simulink library "ComponentLibrary"  (R2017b)
settings: Solver=VariableStepAuto  StartTime=0.0  StopTime=10.0  RelTol=1e-3
undefined symbols (not defined in the file): pelvisPosition, pelvisVelocity, X, Y, Z
libraries: xpcethercatlib x79, sm_lib x21, nesl_utility x13, slrtlib x3, ComponentLibrary x2
(part 1 of 2)
settings Model: Creator=Mikhail  LastModifiedBy=jreher

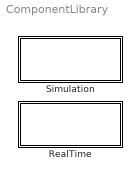
== system ComponentLibrary ==
  RealTime : Subsystem
  Simulation : Subsystem

== system ComponentLibrary/RealTime ==
  Battery : Subsystem
      mask Display: image('Battery.png');
  Elmo Drive : Subsystem  mask{ethercatName=Drive (Elmo Drive), slaveAddress=0, gearRatio=1, torqueConstant=1, encoderCounts=2^13, peakCurrentLimit=0}
      mask prompts: ethercatName "EtherCAT Name:"; slaveAddress "Slave Address"; gearRatio "Gear Ratio:"; torqueConstant "Torque Constant:"; encoderCounts "Encoder Counts:"; peakCurrentLimit "Peak Current Limit:"
      mask init:
      | % Set PDO transmit
      | set_param([gcb '/Mode of Operation PDO Transmit'], 'sig_name', [ethercatName '.Outputs.Mode of operation']);
      | set_param([gcb '/Target Torque PDO Transmit'], 'sig_name', [ethercatName '.Outputs.Target Torque']);
      | set_param([gcb '/Control Word PDO Transmit'], 'sig_name', [ethercatName '.Outputs.Control word']);
      | 
      | % Set PDO receive
      | set_param([gcb '/Status Word PDO Receive'], 'sig_name', [ethercatName '.Inputs.Status word']);
      | set_param([gcb '/Position Actual PDO Receive'], 'sig_name', [ethercatName '.Inputs.Position actual value']);
      | set_param([gcb '/Velocity Actual PDO Receive'], 'sig_name', [ethercatName '.Inputs.Velocity actual value']);
      | set_param([gcb '/Torque Actual PDO Receive'], 'sig_name', [ethercatName '.Inputs.Torque actual value']);
      | set_param([gcb '/DC Link Voltage PDO Receive'], 'sig_name', [ethercatName '.Inputs.DC link circuit voltage']);
      | 
      | % Set SDO temperature upload
      | set_param([gcb '/Drive Temperature Sync SDO Upload'], 'index', '8867');
      | set_param([gcb '/Drive Temperature Sync SDO Upload'], 'subIndex', '1');
      | set_param([gcb '/Drive Temperature Sync SDO Upload'], 'slave_name', ethercatName);
      | set_param([gcb '/Drive Temperature Sync SDO Upload'], 'slave_addr', num2str(slaveAddress));
      | set_param([gcb '/Drive Temperature Sync SDO Upload'], 'slave_found', '1');
      | 
      | % Set SDO Current limit upload
      | set_param([gcb '/Current Limit Sync SDO Upload'], 'index', '12351');
      | set_param([gcb '/Current Limit Sync SDO Upload'], 'subIndex', '1');
      | set_param([gcb '/Current Limit Sync SDO Upload'], 'slave_name', ethercatName);
      | set_param([gcb '/Current Limit Sync SDO Upload'], 'slave_addr', num2str(slaveAddress));
      | set_param([gcb '/Current Limit Sync SDO Upload'], 'slave_found', '1');
      mask Display: image('Elmo Drive.png')
  Radio : Subsystem
      mask Display: image('Radio.png');
  Target PC : Subsystem  mask{config_file=, pci_bus=0, pci_slot=0, pci_function=0}
      mask prompts: config_file "EtherCAT configuration file:"; pci_bus "PCI bus:"; pci_slot "PCI slot:"; pci_function "PCI function:"
      mask TypeOptions config_file: EtherCAT Init/config_file
      mask TypeOptions pci_bus: EtherCAT Init/pci_bus
      mask TypeOptions pci_slot: EtherCAT Init/pci_slot
      mask TypeOptions pci_function: EtherCAT Init/pci_function
  VectorNav : Subsystem  mask{preRotationMatrix=eye(3), postRotationMatrix=eye(3)}
      mask prompts: preRotationMatrix "Pre Rotation Matrix:"; postRotationMatrix "Post Rotation Matrix:"
      mask Display: image('VectorNav.png')

== system ComponentLibrary/Simulation ==
  Battery : Subsystem
      mask Display: image('Battery.png');
  Elmo Drive : Subsystem  mask{gearRatio=25, rotorInertia=0.000061, encoderResolution=2^13, peakTorque=4.5, peakSpeed=2900*(2*pi/60), initialPosition=0, initialVelocity=0}
      mask prompts: gearRatio "Gear Ratio:"; rotorInertia "Motor rotor inertia (kg*m^2):"; encoderResolution "Input Encoder Resolution (ticks/rev):"; peakTorque "Peak torque of motor (N*m):"; peakSpeed "Peak speed of motor (rad/s):"; initialPosition "Initial Position (rad):"; initialVelocity "Initial Velocity (rad/s):"
      mask Display: image('Elmo Drive.png');
  Radio : Subsystem
      mask Display: image('Radio.png');
  Target PC : Subsystem
  VectorNav : Subsystem  mask{preRotationMatrix=eye(3), postRotationMatrix=eye(3)}
      mask prompts: preRotationMatrix "Pre Rotation Matrix:"; postRotationMatrix "Post Rotation Matrix"
      mask Display: image('VectorNav.png');
  World : Subsystem

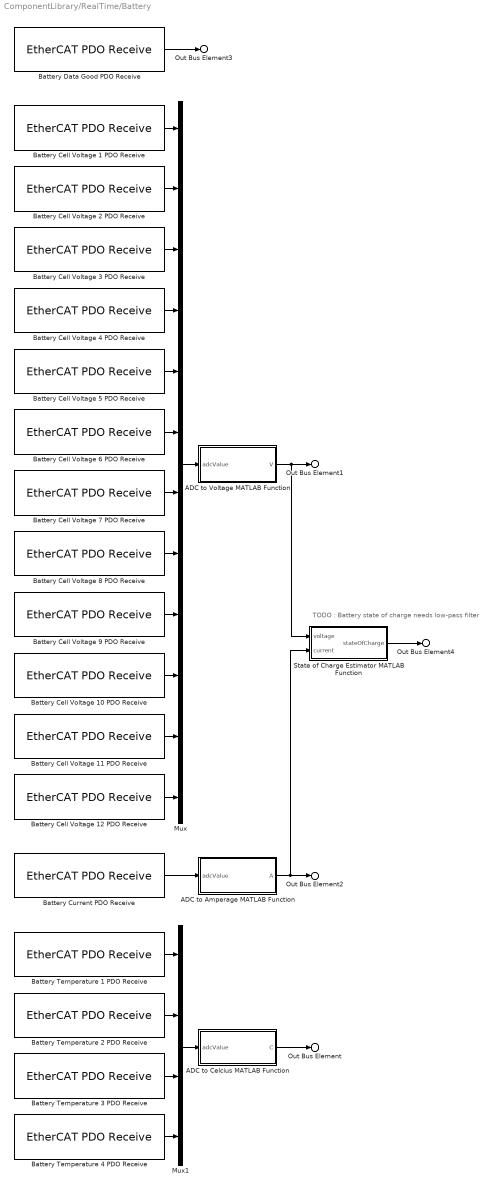
== system ComponentLibrary/RealTime/Battery ==
  note: TODO : Battery state of charge needs low-pass filter
  ADC to Amperage MATLAB Function : MATLAB Function  TreatAsAtomicUnit=on
  ADC to Celcius MATLAB Function : MATLAB Function  TreatAsAtomicUnit=on
  ADC to Voltage MATLAB Function : MATLAB Function  TreatAsAtomicUnit=on
  Battery Cell Voltage 1 PDO Receive : xpcethercatlib/EtherCAT PDO Receive  Priority=2  sig_name=Pelvis Medulla.BMS Inputs.Cell Voltage 01  sig_offset=1608  sig_type=uint16  type_size=16  sig_dim=1  device_id=0  sample_time=0.000500
      settings: SourceProductName=Simulink Real-Time  SourceProductBaseCode=XP
  Battery Cell Voltage 10 PDO Receive : xpcethercatlib/EtherCAT PDO Receive  Priority=2  sig_name=Pelvis Medulla.BMS Inputs.Cell Voltage 10  sig_offset=1752  sig_type=uint16  type_size=16  sig_dim=1  device_id=0  sample_time=0.000500
      settings: SourceProductName=Simulink Real-Time  SourceProductBaseCode=XP
  Battery Cell Voltage 11 PDO Receive : xpcethercatlib/EtherCAT PDO Receive  Priority=2  sig_name=Pelvis Medulla.BMS Inputs.Cell Voltage 11  sig_offset=1768  sig_type=uint16  type_size=16  sig_dim=1  device_id=0  sample_time=0.000500
      settings: SourceProductName=Simulink Real-Time  SourceProductBaseCode=XP
  Battery Cell Voltage 12 PDO Receive : xpcethercatlib/EtherCAT PDO Receive  Priority=2  sig_name=Pelvis Medulla.BMS Inputs.Cell Voltage 12  sig_offset=1784  sig_type=uint16  type_size=16  sig_dim=1  device_id=0  sample_time=0.000500
      settings: SourceProductName=Simulink Real-Time  SourceProductBaseCode=XP
  Battery Cell Voltage 2 PDO Receive : xpcethercatlib/EtherCAT PDO Receive  Priority=2  sig_name=Pelvis Medulla.BMS Inputs.Cell Voltage 02  sig_offset=1624  sig_type=uint16  type_size=16  sig_dim=1  device_id=0  sample_time=0.000500
      settings: SourceProductName=Simulink Real-Time  SourceProductBaseCode=XP
  Battery Cell Voltage 3 PDO Receive : xpcethercatlib/EtherCAT PDO Receive  Priority=2  sig_name=Pelvis Medulla.BMS Inputs.Cell Voltage 03  sig_offset=1640  sig_type=uint16  type_size=16  sig_dim=1  device_id=0  sample_time=0.000500
      settings: SourceProductName=Simulink Real-Time  SourceProductBaseCode=XP
  Battery Cell Voltage 4 PDO Receive : xpcethercatlib/EtherCAT PDO Receive  Priority=2  sig_name=Pelvis Medulla.BMS Inputs.Cell Voltage 04  sig_offset=1656  sig_type=uint16  type_size=16  sig_dim=1  device_id=0  sample_time=0.000500
      settings: SourceProductName=Simulink Real-Time  SourceProductBaseCode=XP
  Battery Cell Voltage 5 PDO Receive : xpcethercatlib/EtherCAT PDO Receive  Priority=2  sig_name=Pelvis Medulla.BMS Inputs.Cell Voltage 05  sig_offset=1672  sig_type=uint16  type_size=16  sig_dim=1  device_id=0  sample_time=0.000500
      settings: SourceProductName=Simulink Real-Time  SourceProductBaseCode=XP
  Battery Cell Voltage 6 PDO Receive : xpcethercatlib/EtherCAT PDO Receive  Priority=2  sig_name=Pelvis Medulla.BMS Inputs.Cell Voltage 06  sig_offset=1688  sig_type=uint16  type_size=16  sig_dim=1  device_id=0  sample_time=0.000500
      settings: SourceProductName=Simulink Real-Time  SourceProductBaseCode=XP
  Battery Cell Voltage 7 PDO Receive : xpcethercatlib/EtherCAT PDO Receive  Priority=2  sig_name=Pelvis Medulla.BMS Inputs.Cell Voltage 07  sig_offset=1704  sig_type=uint16  type_size=16  sig_dim=1  device_id=0  sample_time=0.000500
      settings: SourceProductName=Simulink Real-Time  SourceProductBaseCode=XP
  Battery Cell Voltage 8 PDO Receive : xpcethercatlib/EtherCAT PDO Receive  Priority=2  sig_name=Pelvis Medulla.BMS Inputs.Cell Voltage 08  sig_offset=1720  sig_type=uint16  type_size=16  sig_dim=1  device_id=0  sample_time=0.000500
      settings: SourceProductName=Simulink Real-Time  SourceProductBaseCode=XP
  Battery Cell Voltage 9 PDO Receive : xpcethercatlib/EtherCAT PDO Receive  Priority=2  sig_name=Pelvis Medulla.BMS Inputs.Cell Voltage 09  sig_offset=1736  sig_type=uint16  type_size=16  sig_dim=1  device_id=0  sample_time=0.000500
      settings: SourceProductName=Simulink Real-Time  SourceProductBaseCode=XP
  Battery Current PDO Receive : xpcethercatlib/EtherCAT PDO Receive  Priority=2  sig_name=Pelvis Medulla.BMS Inputs.Current  sig_offset=1864  sig_type=uint16  type_size=16  sig_dim=1  device_id=0  sample_time=0.000500
      settings: SourceProductName=Simulink Real-Time  SourceProductBaseCode=XP
  Battery Data Good PDO Receive : xpcethercatlib/EtherCAT PDO Receive  Priority=2  sig_name=Pelvis Medulla.BMS Inputs.Battery Data Good  sig_offset=1816  sig_type=boolean  type_size=1  sig_dim=1  device_id=0  sample_time=0.0005
      settings: SourceProductName=Simulink Real-Time  SourceProductBaseCode=XP
  Battery Temperature 1 PDO Receive : xpcethercatlib/EtherCAT PDO Receive  Priority=2  sig_name=Pelvis Medulla.BMS Inputs.Temperature 1  sig_offset=1800  sig_type=uint16  type_size=16  sig_dim=1  device_id=0  sample_time=0.000500
      settings: SourceProductName=Simulink Real-Time  SourceProductBaseCode=XP
  Battery Temperature 2 PDO Receive : xpcethercatlib/EtherCAT PDO Receive  Priority=2  sig_name=Pelvis Medulla.BMS Inputs.Temperature 2  sig_offset=1816  sig_type=uint16  type_size=16  sig_dim=1  device_id=0  sample_time=0.000500
      settings: SourceProductName=Simulink Real-Time  SourceProductBaseCode=XP
  Battery Temperature 3 PDO Receive : xpcethercatlib/EtherCAT PDO Receive  Priority=2  sig_name=Pelvis Medulla.BMS Inputs.Temperature 3  sig_offset=1832  sig_type=uint16  type_size=16  sig_dim=1  device_id=0  sample_time=0.000500
      settings: SourceProductName=Simulink Real-Time  SourceProductBaseCode=XP
  Battery Temperature 4 PDO Receive : xpcethercatlib/EtherCAT PDO Receive  Priority=2  sig_name=Pelvis Medulla.BMS Inputs.Temperature 4  sig_offset=1848  sig_type=uint16  type_size=16  sig_dim=1  device_id=0  sample_time=0.000500
      settings: SourceProductName=Simulink Real-Time  SourceProductBaseCode=XP
  Mux : Mux  Inputs=12
  Mux1 : Mux
  State of Charge Estimator MATLAB Function : MATLAB Function  TreatAsAtomicUnit=on
  Out Bus Element3 : Outport  PortName=OutBus  Element=dataGood
  Out Bus Element4 : Outport  PortName=OutBus  Element=stateOfCharge
  Out Bus Element1 : Outport  PortName=OutBus  Element=voltage
  Out Bus Element2 : Outport  PortName=OutBus  Element=current
  Out Bus Element : Outport  PortName=OutBus  Element=temperature
  wires:
  Battery Temperature 1 PDO Receive/1 -> Mux1/1
  Battery Temperature 2 PDO Receive/1 -> Mux1/2
  Battery Temperature 3 PDO Receive/1 -> Mux1/3
  Battery Temperature 4 PDO Receive/1 -> Mux1/4
  Battery Cell Voltage 1 PDO Receive/1 -> Mux/1
  Battery Cell Voltage 2 PDO Receive/1 -> Mux/2
  Battery Cell Voltage 3 PDO Receive/1 -> Mux/3
  Battery Cell Voltage 4 PDO Receive/1 -> Mux/4
  Battery Cell Voltage 5 PDO Receive/1 -> Mux/5
  Battery Cell Voltage 6 PDO Receive/1 -> Mux/6
  Battery Cell Voltage 7 PDO Receive/1 -> Mux/7
  Battery Cell Voltage 8 PDO Receive/1 -> Mux/8
  Battery Cell Voltage 9 PDO Receive/1 -> Mux/9
  Battery Cell Voltage 10 PDO Receive/1 -> Mux/10
  Battery Cell Voltage 11 PDO Receive/1 -> Mux/11
  Battery Cell Voltage 12 PDO Receive/1 -> Mux/12
  Mux/1 -> ADC to Voltage MATLAB Function/1(adcValue)
  Battery Current PDO Receive/1 -> ADC to Amperage MATLAB Function/1(adcValue)
  ADC to Celcius MATLAB Function/1(C) -> Out Bus Element/1
  ADC to Voltage MATLAB Function/1(V) -> State of Charge Estimator MATLAB Function/1(voltage), Out Bus Element1/1
  ADC to Amperage MATLAB Function/1(A) -> State of Charge Estimator MATLAB Function/2(current), Out Bus Element2/1
  Battery Data Good PDO Receive/1 -> Out Bus Element3/1
  Mux1/1 -> ADC to Celcius MATLAB Function/1(adcValue)
  State of Charge Estimator MATLAB Function/1(stateOfCharge) -> Out Bus Element4/1

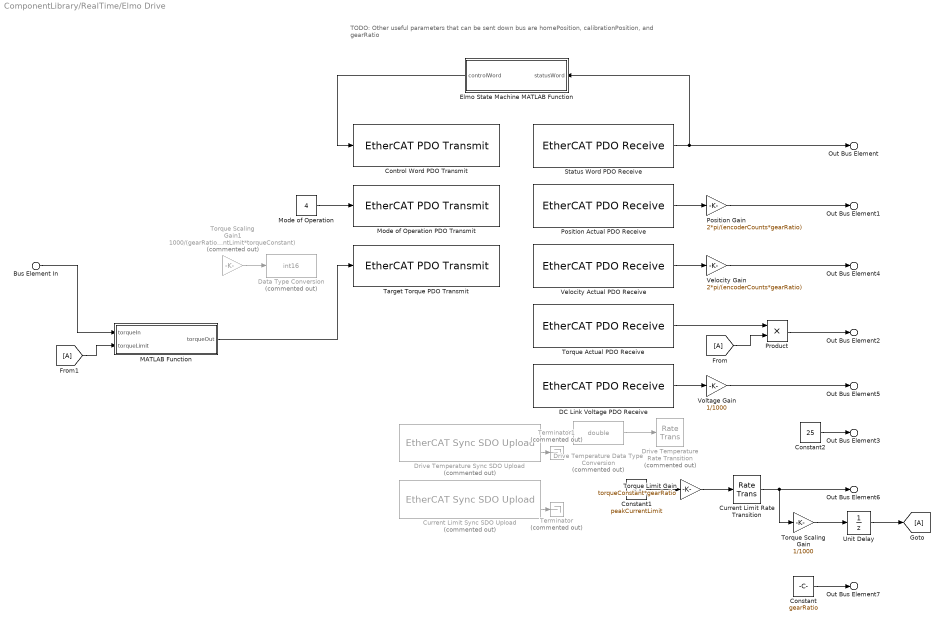
== system ComponentLibrary/RealTime/Elmo Drive ==
  note: TODO: Other useful parameters that can be sent down bus are homePosition, calibrationPosition, and gearRatio
  Bus Element In : Inport  PortName=InBus  Element=torque
  Constant : Constant  Value=gearRatio
  Constant1 : Constant  Value=peakCurrentLimit
  Constant2 : Constant  Value=25
  Control Word PDO Transmit : xpcethercatlib/EtherCAT PDO Transmit   Priority=3  sig_name=Drive (Elmo Drive).Outputs.Control word  sig_offset=2144  sig_type=uint16  type_size=16  sig_dim=1  device_id=0  sample_time=0.001000
      settings: SourceProductName=Simulink Real-Time  SourceProductBaseCode=XP
  Current Limit Rate Transition : RateTransition  Priority=25
  Current Limit Sync SDO Upload : xpcethercatlib/EtherCAT Sync SDO Upload  Priority=25  Commented=on  index=12351  subIndex=1  sig_type=single  sig_dim=1  device_id=0  slave_name=Drive (Elmo Drive)  sample_time=1  slave_addr=0  selected_slave=Term 1 (EK1100)  timeout=50  slave_found=1
      settings: SourceProductName=Simulink Real-Time  SourceProductBaseCode=XP
  DC Link Voltage PDO Receive : xpcethercatlib/EtherCAT PDO Receive  Priority=2  sig_name=Drive (Elmo Drive).Inputs.DC link circuit voltage  sig_offset=2128  sig_type=int32  type_size=32  sig_dim=1  device_id=0  sample_time=0.001000
      settings: SourceProductName=Simulink Real-Time  SourceProductBaseCode=XP
  Data Type Conversion : DataTypeConversion  Commented=on  OutDataTypeStr=int16
  Drive Temperature Data Type Conversion : DataTypeConversion  Priority=25  Commented=on  OutDataTypeStr=double
  Drive Temperature Rate Transition : RateTransition  Priority=25  Commented=on
  Drive Temperature Sync SDO Upload : xpcethercatlib/EtherCAT Sync SDO Upload  Priority=25  Commented=on  index=8867  subIndex=1  sig_type=uint16  sig_dim=1  device_id=0  slave_name=Drive (Elmo Drive)  sample_time=1  slave_addr=0  selected_slave=Term 1 (EK1100)  timeout=50  slave_found=1
      settings: SourceProductName=Simulink Real-Time  SourceProductBaseCode=XP
  Elmo State Machine MATLAB Function : MATLAB Function  TreatAsAtomicUnit=on
  MATLAB Function : MATLAB Function  TreatAsAtomicUnit=on
  Mode of Operation : Constant  Value=4  OutDataTypeStr=int8
  Mode of Operation PDO Transmit : xpcethercatlib/EtherCAT PDO Transmit   Priority=3  sig_name=Drive (Elmo Drive).Outputs.Mode of operation  sig_offset=2160  sig_type=int8  type_size=8  sig_dim=1  device_id=0  sample_time=0.001000
      settings: SourceProductName=Simulink Real-Time  SourceProductBaseCode=XP
  Position Gain : Gain  Gain=2*pi/(encoderCounts*gearRatio)  ParamDataTypeStr=double  OutDataTypeStr=double
  Position Actual PDO Receive : xpcethercatlib/EtherCAT PDO Receive  Priority=2  sig_name=Drive (Elmo Drive).Inputs.Position actual value  sig_offset=2128  sig_type=int32  type_size=32  sig_dim=1  device_id=0  sample_time=0.001000
      settings: SourceProductName=Simulink Real-Time  SourceProductBaseCode=XP
  Product : Product  OutDataTypeStr=double
  Status Word PDO Receive : xpcethercatlib/EtherCAT PDO Receive  Priority=2  sig_name=Drive (Elmo Drive).Inputs.Status word  sig_offset=2176  sig_type=uint16  type_size=16  sig_dim=1  device_id=0  sample_time=0.001000
      settings: SourceProductName=Simulink Real-Time  SourceProductBaseCode=XP
  Target Torque PDO Transmit : xpcethercatlib/EtherCAT PDO Transmit   Priority=3  sig_name=Drive (Elmo Drive).Outputs.Target Torque  sig_offset=2128  sig_type=int16  type_size=16  sig_dim=1  device_id=0  sample_time=0.001000
      settings: SourceProductName=Simulink Real-Time  SourceProductBaseCode=XP
  Terminator : Terminator  Commented=on
  Terminator1 : Terminator  Commented=on
  Torque Actual PDO Receive : xpcethercatlib/EtherCAT PDO Receive  Priority=2  sig_name=Drive (Elmo Drive).Inputs.Torque actual value  sig_offset=2128  sig_type=int32  type_size=32  sig_dim=1  device_id=0  sample_time=0.001000
      settings: SourceProductName=Simulink Real-Time  SourceProductBaseCode=XP
  Torque Limit Gain : Gain  Priority=25  Gain=torqueConstant*gearRatio  OutDataTypeStr=double
  Torque Scaling Gain : Gain  Gain=1/1000  ParamDataTypeStr=double  OutDataTypeStr=double
  Torque Scaling Gain1 : Gain  Commented=on  Gain=1000/(gearRatio*peakCurrentLimit*torqueConstant)  ParamDataTypeStr=double  OutDataTypeStr=double
  Unit Delay : UnitDelay  InitialCondition=1  SampleTime=-1
  Velocity Gain : Gain  Gain=2*pi/(encoderCounts*gearRatio)  ParamDataTypeStr=double  OutDataTypeStr=double
  Velocity Actual PDO Receive : xpcethercatlib/EtherCAT PDO Receive  Priority=2  sig_name=Drive (Elmo Drive).Inputs.Velocity actual value  sig_offset=2128  sig_type=int32  type_size=32  sig_dim=1  device_id=0  sample_time=0.001000
      settings: SourceProductName=Simulink Real-Time  SourceProductBaseCode=XP
  Voltage Gain : Gain  Gain=1/1000  ParamDataTypeStr=double  OutDataTypeStr=double
  Out Bus Element : Outport  PortName=OutBus  Element=statusWord
  Out Bus Element1 : Outport  PortName=OutBus  Element=position
  Out Bus Element4 : Outport  PortName=OutBus  Element=velocity
  Out Bus Element2 : Outport  PortName=OutBus  Element=torque
  Out Bus Element3 : Outport  PortName=OutBus  Element=driveTemperature
  Out Bus Element5 : Outport  PortName=OutBus  Element=dcLinkVoltage
  Out Bus Element6 : Outport  PortName=OutBus  Element=torqueLimit
  Out Bus Element7 : Outport  PortName=OutBus  Element=gearRatio
  wires:
  Position Actual PDO Receive/1 -> Position Gain/1
  Mode of Operation/1 -> Mode of Operation PDO Transmit/1
  Status Word PDO Receive/1 -> Elmo State Machine MATLAB Function/1(statusWord), Out Bus Element/1
  Elmo State Machine MATLAB Function/1(controlWord) -> Control Word PDO Transmit/1
  Torque Actual PDO Receive/1 -> Product/1
  Drive Temperature Data Type Conversion/1 -> Drive Temperature Rate Transition/1
  Position Gain/1 -> Out Bus Element1/1
  Product/1 -> Out Bus Element2/1
  DC Link Voltage PDO Receive/1 -> Voltage Gain/1
  Voltage Gain/1 -> Out Bus Element5/1
  Velocity Gain/1 -> Out Bus Element4/1
  Velocity Actual PDO Receive/1 -> Velocity Gain/1
  Drive Temperature Sync SDO Upload/1 -> Drive Temperature Data Type Conversion/1
  Torque Limit Gain/1 -> Current Limit Rate Transition/1
  Current Limit Rate Transition/1 -> Torque Scaling Gain/1, Out Bus Element6/1
  Current Limit Sync SDO Upload/2 -> Terminator/1
  Drive Temperature Sync SDO Upload/2 -> Terminator1/1
  Torque Scaling Gain/1 -> Unit Delay/1
  Unit Delay/1 -> [A]
  [A] -> Product/2
  Constant/1 -> Out Bus Element7/1
  [A] -> MATLAB Function/2(torqueLimit)
  Torque Scaling Gain1/1 -> Data Type Conversion/1
  Bus Element In/1 -> MATLAB Function/1(torqueIn)
  MATLAB Function/1(torqueOut) -> Target Torque PDO Transmit/1
  Constant2/1 -> Out Bus Element3/1
  Constant1/1 -> Torque Limit Gain/1

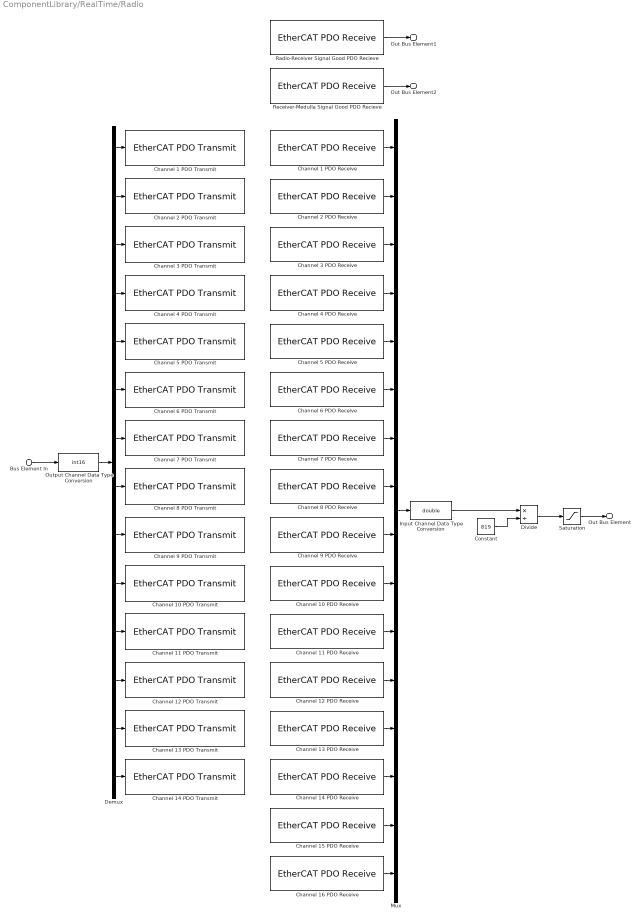
== system ComponentLibrary/RealTime/Radio ==
  Bus Element In : Inport  PortName=InBus  Element=channel
  Channel 1 PDO Receive : xpcethercatlib/EtherCAT PDO Receive  Priority=2  sig_name=Pelvis Medulla.Radio Inputs.Channel 01  sig_offset=616  sig_type=int16  type_size=16  sig_dim=1  device_id=0  sample_time=0.000500
      settings: SourceProductName=Simulink Real-Time  SourceProductBaseCode=XP
  Channel 1 PDO Transmit : xpcethercatlib/EtherCAT PDO Transmit   Priority=3  sig_name=Pelvis Medulla.Radio Outputs.Channel 01  sig_offset=592  sig_type=int16  type_size=16  sig_dim=1  device_id=0  sample_time=0.000500
      settings: SourceProductName=Simulink Real-Time  SourceProductBaseCode=XP
  Channel 10 PDO Receive : xpcethercatlib/EtherCAT PDO Receive  Priority=2  sig_name=Pelvis Medulla.Radio Inputs.Channel 10  sig_offset=760  sig_type=int16  type_size=16  sig_dim=1  device_id=0  sample_time=0.000500
      settings: SourceProductName=Simulink Real-Time  SourceProductBaseCode=XP
  Channel 10 PDO Transmit : xpcethercatlib/EtherCAT PDO Transmit   Priority=3  sig_name=Pelvis Medulla.Radio Outputs.Channel 10  sig_offset=736  sig_type=int16  type_size=16  sig_dim=1  device_id=0  sample_time=0.000500
      settings: SourceProductName=Simulink Real-Time  SourceProductBaseCode=XP
  Channel 11 PDO Receive : xpcethercatlib/EtherCAT PDO Receive  Priority=2  sig_name=Pelvis Medulla.Radio Inputs.Channel 11  sig_offset=776  sig_type=int16  type_size=16  sig_dim=1  device_id=0  sample_time=0.000500
      settings: SourceProductName=Simulink Real-Time  SourceProductBaseCode=XP
  Channel 11 PDO Transmit : xpcethercatlib/EtherCAT PDO Transmit   Priority=3  sig_name=Pelvis Medulla.Radio Outputs.Channel 11  sig_offset=752  sig_type=int16  type_size=16  sig_dim=1  device_id=0  sample_time=0.000500
      settings: SourceProductName=Simulink Real-Time  SourceProductBaseCode=XP
  Channel 12 PDO Receive : xpcethercatlib/EtherCAT PDO Receive  Priority=2  sig_name=Pelvis Medulla.Radio Inputs.Channel 12  sig_offset=792  sig_type=int16  type_size=16  sig_dim=1  device_id=0  sample_time=0.000500
      settings: SourceProductName=Simulink Real-Time  SourceProductBaseCode=XP
  Channel 12 PDO Transmit : xpcethercatlib/EtherCAT PDO Transmit   Priority=3  sig_name=Pelvis Medulla.Radio Outputs.Channel 12  sig_offset=768  sig_type=int16  type_size=16  sig_dim=1  device_id=0  sample_time=0.000500
      settings: SourceProductName=Simulink Real-Time  SourceProductBaseCode=XP
  Channel 13 PDO Receive : xpcethercatlib/EtherCAT PDO Receive  Priority=2  sig_name=Pelvis Medulla.Radio Inputs.Channel 13  sig_offset=808  sig_type=int16  type_size=16  sig_dim=1  device_id=0  sample_time=0.000500
      settings: SourceProductName=Simulink Real-Time  SourceProductBaseCode=XP
  Channel 13 PDO Transmit : xpcethercatlib/EtherCAT PDO Transmit   Priority=3  sig_name=Pelvis Medulla.Radio Outputs.Channel 13  sig_offset=784  sig_type=int16  type_size=16  sig_dim=1  device_id=0  sample_time=0.000500
      settings: SourceProductName=Simulink Real-Time  SourceProductBaseCode=XP
  Channel 14 PDO Receive : xpcethercatlib/EtherCAT PDO Receive  Priority=2  sig_name=Pelvis Medulla.Radio Inputs.Channel 14  sig_offset=824  sig_type=int16  type_size=16  sig_dim=1  device_id=0  sample_time=0.000500
      settings: SourceProductName=Simulink Real-Time  SourceProductBaseCode=XP
  Channel 14 PDO Transmit : xpcethercatlib/EtherCAT PDO Transmit   Priority=3  sig_name=Pelvis Medulla.Radio Outputs.Channel 14  sig_offset=800  sig_type=int16  type_size=16  sig_dim=1  device_id=0  sample_time=0.000500
      settings: SourceProductName=Simulink Real-Time  SourceProductBaseCode=XP
  Channel 15 PDO Receive : xpcethercatlib/EtherCAT PDO Receive  Priority=2  sig_name=Pelvis Medulla.Radio Inputs.Channel 15  sig_offset=840  sig_type=int16  type_size=16  sig_dim=1  device_id=0  sample_time=0.000500
      settings: SourceProductName=Simulink Real-Time  SourceProductBaseCode=XP
  Channel 16 PDO Receive : xpcethercatlib/EtherCAT PDO Receive  Priority=2  sig_name=Pelvis Medulla.Radio Inputs.Channel 16  sig_offset=856  sig_type=int16  type_size=16  sig_dim=1  device_id=0  sample_time=0.000500
      settings: SourceProductName=Simulink Real-Time  SourceProductBaseCode=XP
  Channel 2 PDO Receive : xpcethercatlib/EtherCAT PDO Receive  Priority=2  sig_name=Pelvis Medulla.Radio Inputs.Channel 02  sig_offset=632  sig_type=int16  type_size=16  sig_dim=1  device_id=0  sample_time=0.000500
      settings: SourceProductName=Simulink Real-Time  SourceProductBaseCode=XP
  Channel 2 PDO Transmit : xpcethercatlib/EtherCAT PDO Transmit   Priority=3  sig_name=Pelvis Medulla.Radio Outputs.Channel 02  sig_offset=608  sig_type=int16  type_size=16  sig_dim=1  device_id=0  sample_time=0.000500
      settings: SourceProductName=Simulink Real-Time  SourceProductBaseCode=XP
  Channel 3 PDO Receive : xpcethercatlib/EtherCAT PDO Receive  Priority=2  sig_name=Pelvis Medulla.Radio Inputs.Channel 03  sig_offset=648  sig_type=int16  type_size=16  sig_dim=1  device_id=0  sample_time=0.000500
      settings: SourceProductName=Simulink Real-Time  SourceProductBaseCode=XP
  Channel 3 PDO Transmit : xpcethercatlib/EtherCAT PDO Transmit   Priority=3  sig_name=Pelvis Medulla.Radio Outputs.Channel 03  sig_offset=624  sig_type=int16  type_size=16  sig_dim=1  device_id=0  sample_time=0.000500
      settings: SourceProductName=Simulink Real-Time  SourceProductBaseCode=XP
  Channel 4 PDO Receive : xpcethercatlib/EtherCAT PDO Receive  Priority=2  sig_name=Pelvis Medulla.Radio Inputs.Channel 04  sig_offset=664  sig_type=int16  type_size=16  sig_dim=1  device_id=0  sample_time=0.000500
      settings: SourceProductName=Simulink Real-Time  SourceProductBaseCode=XP
  Channel 4 PDO Transmit : xpcethercatlib/EtherCAT PDO Transmit   Priority=3  sig_name=Pelvis Medulla.Radio Outputs.Channel 04  sig_offset=640  sig_type=int16  type_size=16  sig_dim=1  device_id=0  sample_time=0.000500
      settings: SourceProductName=Simulink Real-Time  SourceProductBaseCode=XP
  Channel 5 PDO Receive : xpcethercatlib/EtherCAT PDO Receive  Priority=2  sig_name=Pelvis Medulla.Radio Inputs.Channel 05  sig_offset=680  sig_type=int16  type_size=16  sig_dim=1  device_id=0  sample_time=0.000500
      settings: SourceProductName=Simulink Real-Time  SourceProductBaseCode=XP
  Channel 5 PDO Transmit : xpcethercatlib/EtherCAT PDO Transmit   Priority=3  sig_name=Pelvis Medulla.Radio Outputs.Channel 05  sig_offset=656  sig_type=int16  type_size=16  sig_dim=1  device_id=0  sample_time=0.000500
      settings: SourceProductName=Simulink Real-Time  SourceProductBaseCode=XP
  Channel 6 PDO Receive : xpcethercatlib/EtherCAT PDO Receive  Priority=2  sig_name=Pelvis Medulla.Radio Inputs.Channel 06  sig_offset=696  sig_type=int16  type_size=16  sig_dim=1  device_id=0  sample_time=0.000500
      settings: SourceProductName=Simulink Real-Time  SourceProductBaseCode=XP
  Channel 6 PDO Transmit : xpcethercatlib/EtherCAT PDO Transmit   Priority=3  sig_name=Pelvis Medulla.Radio Outputs.Channel 06  sig_offset=672  sig_type=int16  type_size=16  sig_dim=1  device_id=0  sample_time=0.000500
      settings: SourceProductName=Simulink Real-Time  SourceProductBaseCode=XP
  Channel 7 PDO Receive : xpcethercatlib/EtherCAT PDO Receive  Priority=2  sig_name=Pelvis Medulla.Radio Inputs.Channel 07  sig_offset=712  sig_type=int16  type_size=16  sig_dim=1  device_id=0  sample_time=0.000500
      settings: SourceProductName=Simulink Real-Time  SourceProductBaseCode=XP
  Channel 7 PDO Transmit : xpcethercatlib/EtherCAT PDO Transmit   Priority=3  sig_name=Pelvis Medulla.Radio Outputs.Channel 07  sig_offset=688  sig_type=int16  type_size=16  sig_dim=1  device_id=0  sample_time=0.000500
      settings: SourceProductName=Simulink Real-Time  SourceProductBaseCode=XP
  Channel 8 PDO Receive : xpcethercatlib/EtherCAT PDO Receive  Priority=2  sig_name=Pelvis Medulla.Radio Inputs.Channel 08  sig_offset=728  sig_type=int16  type_size=16  sig_dim=1  device_id=0  sample_time=0.000500
      settings: SourceProductName=Simulink Real-Time  SourceProductBaseCode=XP
  Channel 8 PDO Transmit : xpcethercatlib/EtherCAT PDO Transmit   Priority=3  sig_name=Pelvis Medulla.Radio Outputs.Channel 08  sig_offset=704  sig_type=int16  type_size=16  sig_dim=1  device_id=0  sample_time=0.000500
      settings: SourceProductName=Simulink Real-Time  SourceProductBaseCode=XP
  Channel 9 PDO Receive : xpcethercatlib/EtherCAT PDO Receive  Priority=2  sig_name=Pelvis Medulla.Radio Inputs.Channel 09  sig_offset=744  sig_type=int16  type_size=16  sig_dim=1  device_id=0  sample_time=0.000500
      settings: SourceProductName=Simulink Real-Time  SourceProductBaseCode=XP
  Channel 9 PDO Transmit : xpcethercatlib/EtherCAT PDO Transmit   Priority=3  sig_name=Pelvis Medulla.Radio Outputs.Channel 09  sig_offset=720  sig_type=int16  type_size=16  sig_dim=1  device_id=0  sample_time=0.000500
      settings: SourceProductName=Simulink Real-Time  SourceProductBaseCode=XP
  Constant : Constant  Value=819
  Demux : Demux  Outputs=14
  Divide : Product  Inputs=*/
  Input Channel Data Type Conversion : DataTypeConversion  OutDataTypeStr=double
  Mux : Mux  Inputs=16
  Output Channel Data Type Conversion : DataTypeConversion  OutDataTypeStr=int16
  Radio-Receiver Signal Good PDO Recieve : xpcethercatlib/EtherCAT PDO Receive  Priority=2  sig_name=Pelvis Medulla.Radio Inputs.Radio-Receiver Signal Good  sig_offset=1805  sig_type=boolean  type_size=1  sig_dim=1  device_id=0  sample_time=0.000500
      settings: SourceProductName=Simulink Real-Time  SourceProductBaseCode=XP
  Receiver-Medulla Signal Good PDO Recieve : xpcethercatlib/EtherCAT PDO Receive  Priority=2  sig_name=Pelvis Medulla.Radio Inputs.Receiver-Medulla Signal Good  sig_offset=1806  sig_type=boolean  type_size=1  sig_dim=1  device_id=0  sample_time=0.000500
      settings: SourceProductName=Simulink Real-Time  SourceProductBaseCode=XP
  Saturation : Saturate  UpperLimit=1  LowerLimit=-1
  Out Bus Element1 : Outport  PortName=OutBus  Element=radioReceiverSignalGood
  Out Bus Element2 : Outport  PortName=OutBus  Element=receiverMedullaSignalGood
  Out Bus Element : Outport  PortName=OutBus  Element=channel
  wires:
  Channel 1 PDO Receive/1 -> Mux/1
  Channel 2 PDO Receive/1 -> Mux/2
  Channel 16 PDO Receive/1 -> Mux/16
  Channel 15 PDO Receive/1 -> Mux/15
  Channel 14 PDO Receive/1 -> Mux/14
  Channel 13 PDO Receive/1 -> Mux/13
  Channel 12 PDO Receive/1 -> Mux/12
  Channel 11 PDO Receive/1 -> Mux/11
  Channel 10 PDO Receive/1 -> Mux/10
  Channel 9 PDO Receive/1 -> Mux/9
  Channel 8 PDO Receive/1 -> Mux/8
  Channel 6 PDO Receive/1 -> Mux/6
  Channel 7 PDO Receive/1 -> Mux/7
  Channel 3 PDO Receive/1 -> Mux/3
  Channel 4 PDO Receive/1 -> Mux/4
  Channel 5 PDO Receive/1 -> Mux/5
  Mux/1 -> Input Channel Data Type Conversion/1
  Demux/1 -> Channel 1 PDO Transmit/1
  Demux/14 -> Channel 14 PDO Transmit/1
  Demux/2 -> Channel 2 PDO Transmit/1
  Demux/3 -> Channel 3 PDO Transmit/1
  Demux/4 -> Channel 4 PDO Transmit/1
  Demux/5 -> Channel 5 PDO Transmit/1
  Demux/6 -> Channel 6 PDO Transmit/1
  Demux/7 -> Channel 7 PDO Transmit/1
  Demux/8 -> Channel 8 PDO Transmit/1
  Demux/9 -> Channel 9 PDO Transmit/1
  Demux/10 -> Channel 10 PDO Transmit/1
  Demux/11 -> Channel 11 PDO Transmit/1
  Demux/12 -> Channel 12 PDO Transmit/1
  Demux/13 -> Channel 13 PDO Transmit/1
  Output Channel Data Type Conversion/1 -> Demux/1
  Bus Element In/1 -> Output Channel Data Type Conversion/1
  Radio-Receiver Signal Good PDO Recieve/1 -> Out Bus Element1/1
  Receiver-Medulla Signal Good PDO Recieve/1 -> Out Bus Element2/1
  Constant/1 -> Divide/2
  Divide/1 -> Saturation/1
  Input Channel Data Type Conversion/1 -> Divide/1
  Saturation/1 -> Out Bus Element/1

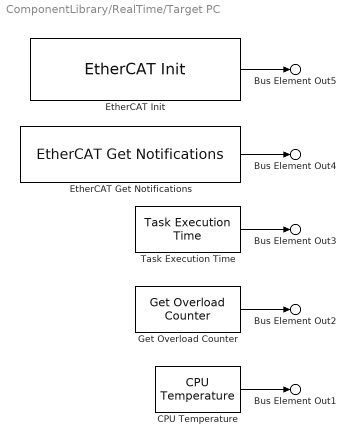
== system ComponentLibrary/RealTime/Target PC ==
  CPU Temperature : slrtlib/Target Management/Target Information/CPU Temperature  ts=-1
      settings: SourceProductName=Simulink Real-Time  SourceProductBaseCode=XP
  EtherCAT Get Notifications : xpcethercatlib/EtherCAT Get Notifications   device_id=0  sample_time=-1
      settings: SourceProductName=Simulink Real-Time  SourceProductBaseCode=XP
  EtherCAT Init : xpcethercatlib/EtherCAT Init   Priority=0  device_id=0  pci_bus=pci_bus  pci_slot=pci_slot  pci_function=pci_function  dctuning=0  enaDebug=off  enaDC=on  errLink=off  masterDbg=off  stateChgDbg=off  baseClock=off  masterCfg=off  logFile='c:\dbglog.txt'  sample_time=0.000500  DCMode=0
      settings: SourceProductName=Simulink Real-Time  SourceProductBaseCode=XP
  Get Overload Counter : slrtlib/Target Management/Execution Parameters/Get Overload Counter   ts=-1
      settings: SourceProductName=Simulink Real-Time  SourceProductBaseCode=XP
  "Task Execution Time " : slrtlib/Target Management/Execution Parameters/Task Execution Time   ts=-1
      settings: SourceProductName=Simulink Real-Time  SourceProductBaseCode=XP
  Bus Element Out5 : Outport  PortName=OutBus  Element=etherCatStatus
  Bus Element Out4 : Outport  PortName=OutBus  Element=etherCatNotifications
  Bus Element Out3 : Outport  PortName=OutBus  Element=taskExecutionTime
  Bus Element Out2 : Outport  PortName=OutBus  Element=overloadCounter
  Bus Element Out1 : Outport  PortName=OutBus  Element=cpuTemperature
  wires:
  CPU Temperature/1 -> Bus Element Out1/1
  "Task Execution Time "/1 -> Bus Element Out3/1
  EtherCAT Get Notifications/1 -> Bus Element Out4/1
  EtherCAT Init/1 -> Bus Element Out5/1
  Get Overload Counter/1 -> Bus Element Out2/1

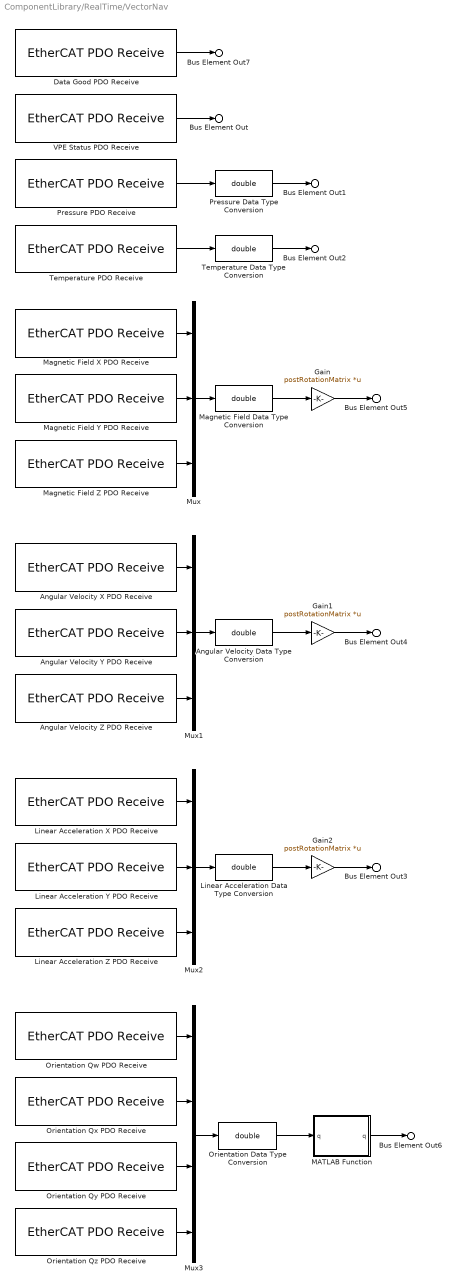
== system ComponentLibrary/RealTime/VectorNav ==
  Angular Velocity Data Type Conversion : DataTypeConversion  OutDataTypeStr=double
  Angular Velocity X PDO Receive : xpcethercatlib/EtherCAT PDO Receive  Priority=2  sig_name=Pelvis Medulla.VN Inputs.Angular Velocity X  sig_offset=1232  sig_type=single  type_size=32  sig_dim=1  device_id=0  sample_time=0.000500
      settings: SourceProductName=Simulink Real-Time  SourceProductBaseCode=XP
  Angular Velocity Y PDO Receive : xpcethercatlib/EtherCAT PDO Receive  Priority=2  sig_name=Pelvis Medulla.VN Inputs.Angular Velocity Y  sig_offset=1264  sig_type=single  type_size=32  sig_dim=1  device_id=0  sample_time=0.000500
      settings: SourceProductName=Simulink Real-Time  SourceProductBaseCode=XP
  Angular Velocity Z PDO Receive : xpcethercatlib/EtherCAT PDO Receive  Priority=2  sig_name=Pelvis Medulla.VN Inputs.Angular Velocity Z  sig_offset=1296  sig_type=single  type_size=32  sig_dim=1  device_id=0  sample_time=0.000500
      settings: SourceProductName=Simulink Real-Time  SourceProductBaseCode=XP
  Data Good PDO Receive : xpcethercatlib/EtherCAT PDO Receive  Priority=2  sig_name=Pelvis Medulla.VN Inputs.VN Data Good  sig_offset=1600  sig_type=boolean  type_size=1  sig_dim=1  device_id=0  sample_time=0.0005
      settings: SourceProductName=Simulink Real-Time  SourceProductBaseCode=XP
  Gain : Gain  Gain=postRotationMatrix  Multiplication=Matrix(K*u)
  Gain1 : Gain  Gain=postRotationMatrix  Multiplication=Matrix(K*u)
  Gain2 : Gain  Gain=postRotationMatrix  Multiplication=Matrix(K*u)
  Linear Acceleration Data Type Conversion : DataTypeConversion  OutDataTypeStr=double
  Linear Acceleration X PDO Receive : xpcethercatlib/EtherCAT PDO Receive  Priority=2  sig_name=Pelvis Medulla.VN Inputs.Linear Acceleration X  sig_offset=1264  sig_type=single  type_size=32  sig_dim=1  device_id=0  sample_time=0.000500
      settings: SourceProductName=Simulink Real-Time  SourceProductBaseCode=XP
  Linear Acceleration Y PDO Receive : xpcethercatlib/EtherCAT PDO Receive  Priority=2  sig_name=Pelvis Medulla.VN Inputs.Linear Acceleration Y  sig_offset=1296  sig_type=single  type_size=32  sig_dim=1  device_id=0  sample_time=0.000500
      settings: SourceProductName=Simulink Real-Time  SourceProductBaseCode=XP
  Linear Acceleration Z PDO Receive : xpcethercatlib/EtherCAT PDO Receive  Priority=2  sig_name=Pelvis Medulla.VN Inputs.Linear Acceleration Z  sig_offset=1328  sig_type=single  type_size=32  sig_dim=1  device_id=0  sample_time=0.000500
      settings: SourceProductName=Simulink Real-Time  SourceProductBaseCode=XP
  MATLAB Function : MATLAB Function  TreatAsAtomicUnit=on
  Magnetic Field Data Type Conversion : DataTypeConversion  OutDataTypeStr=double
  Magnetic Field X PDO Receive : xpcethercatlib/EtherCAT PDO Receive  Priority=2  sig_name=Pelvis Medulla.VN Inputs.Magnetic Field X  sig_offset=1360  sig_type=single  type_size=32  sig_dim=1  device_id=0  sample_time=0.000500
      settings: SourceProductName=Simulink Real-Time  SourceProductBaseCode=XP
  Magnetic Field Y PDO Receive : xpcethercatlib/EtherCAT PDO Receive  Priority=2  sig_name=Pelvis Medulla.VN Inputs.Magnetic Field Y  sig_offset=1392  sig_type=single  type_size=32  sig_dim=1  device_id=0  sample_time=0.000500
      settings: SourceProductName=Simulink Real-Time  SourceProductBaseCode=XP
  Magnetic Field Z PDO Receive : xpcethercatlib/EtherCAT PDO Receive  Priority=2  sig_name=Pelvis Medulla.VN Inputs.Magnetic Field Z  sig_offset=1424  sig_type=single  type_size=32  sig_dim=1  device_id=0  sample_time=0.000500
      settings: SourceProductName=Simulink Real-Time  SourceProductBaseCode=XP
  Mux : Mux  Inputs=3
  Mux1 : Mux  Inputs=3
  Mux2 : Mux  Inputs=3
  Mux3 : Mux
  Orientation Data Type Conversion : DataTypeConversion  OutDataTypeStr=double
  Orientation Qw PDO Receive : xpcethercatlib/EtherCAT PDO Receive  Priority=2  sig_name=Pelvis Medulla.VN Inputs.Orientation Qw  sig_offset=1136  sig_type=single  type_size=32  sig_dim=1  device_id=0  sample_time=0.000500
      settings: SourceProductName=Simulink Real-Time  SourceProductBaseCode=XP
  Orientation Qx PDO Receive : xpcethercatlib/EtherCAT PDO Receive  Priority=2  sig_name=Pelvis Medulla.VN Inputs.Orientation Qx  sig_offset=1040  sig_type=single  type_size=32  sig_dim=1  device_id=0  sample_time=0.000500
      settings: SourceProductName=Simulink Real-Time  SourceProductBaseCode=XP
  Orientation Qy PDO Receive : xpcethercatlib/EtherCAT PDO Receive  Priority=2  sig_name=Pelvis Medulla.VN Inputs.Orientation Qy  sig_offset=1072  sig_type=single  type_size=32  sig_dim=1  device_id=0  sample_time=0.000500
      settings: SourceProductName=Simulink Real-Time  SourceProductBaseCode=XP
  Orientation Qz PDO Receive : xpcethercatlib/EtherCAT PDO Receive  Priority=2  sig_name=Pelvis Medulla.VN Inputs.Orientation Qz  sig_offset=1104  sig_type=single  type_size=32  sig_dim=1  device_id=0  sample_time=0.000500
      settings: SourceProductName=Simulink Real-Time  SourceProductBaseCode=XP
  Pressure Data Type Conversion : DataTypeConversion  OutDataTypeStr=double
  Pressure PDO Receive : xpcethercatlib/EtherCAT PDO Receive  Priority=2  sig_name=Pelvis Medulla.VN Inputs.Pressure  sig_offset=1488  sig_type=single  type_size=32  sig_dim=1  device_id=0  sample_time=0.000500
      settings: SourceProductName=Simulink Real-Time  SourceProductBaseCode=XP
  Temperature Data Type Conversion : DataTypeConversion  OutDataTypeStr=double
  Temperature PDO Receive : xpcethercatlib/EtherCAT PDO Receive  Priority=2  sig_name=Pelvis Medulla.VN Inputs.Temperature  sig_offset=1456  sig_type=single  type_size=32  sig_dim=1  device_id=0  sample_time=0.000500
      settings: SourceProductName=Simulink Real-Time  SourceProductBaseCode=XP
  VPE Status PDO Receive : xpcethercatlib/EtherCAT PDO Receive  Priority=2  sig_name=Pelvis Medulla.VN Inputs.VPE Status  sig_offset=1520  sig_type=uint16  type_size=16  sig_dim=1  device_id=0  sample_time=0.000500
      settings: SourceProductName=Simulink Real-Time  SourceProductBaseCode=XP
  Bus Element Out7 : Outport  PortName=OutBus  Element=dataGood
  Bus Element Out : Outport  PortName=OutBus  Element=vpeStatus
  Bus Element Out1 : Outport  PortName=OutBus  Element=pressure
  Bus Element Out2 : Outport  PortName=OutBus  Element=temperature
  Bus Element Out5 : Outport  PortName=OutBus  Element=magneticField
  Bus Element Out4 : Outport  PortName=OutBus  Element=angularVelocity
  Bus Element Out3 : Outport  PortName=OutBus  Element=linearAcceleration
  Bus Element Out6 : Outport  PortName=OutBus  Element=orientation
  wires:
  Orientation Qw PDO Receive/1 -> Mux3/1
  Magnetic Field X PDO Receive/1 -> Mux/1
  Orientation Qy PDO Receive/1 -> Mux3/3
  Mux2/1 -> Linear Acceleration Data Type Conversion/1
  Mux3/1 -> Orientation Data Type Conversion/1
  Angular Velocity Z PDO Receive/1 -> Mux1/3
  Mux/1 -> Magnetic Field Data Type Conversion/1
  Mux1/1 -> Angular Velocity Data Type Conversion/1
  Angular Velocity Data Type Conversion/1 -> Gain1/1
  Pressure Data Type Conversion/1 -> Bus Element Out1/1
  Angular Velocity Y PDO Receive/1 -> Mux1/2
  Linear Acceleration Y PDO Receive/1 -> Mux2/2
  Pressure PDO Receive/1 -> Pressure Data Type Conversion/1
  VPE Status PDO Receive/1 -> Bus Element Out/1
  Orientation Data Type Conversion/1 -> MATLAB Function/1("q ")
  Orientation Qz PDO Receive/1 -> Mux3/4
  Data Good PDO Receive/1 -> Bus Element Out7/1
  Magnetic Field Data Type Conversion/1 -> Gain/1
  Orientation Qx PDO Receive/1 -> Mux3/2
  Angular Velocity X PDO Receive/1 -> Mux1/1
  Magnetic Field Z PDO Receive/1 -> Mux/3
  Linear Acceleration X PDO Receive/1 -> Mux2/1
  Temperature Data Type Conversion/1 -> Bus Element Out2/1
  Linear Acceleration Data Type Conversion/1 -> Gain2/1
  Magnetic Field Y PDO Receive/1 -> Mux/2
  Linear Acceleration Z PDO Receive/1 -> Mux2/3
  Temperature PDO Receive/1 -> Temperature Data Type Conversion/1
  Gain/1 -> Bus Element Out5/1
  Gain1/1 -> Bus Element Out4/1
  Gain2/1 -> Bus Element Out3/1
  MATLAB Function/1(q) -> Bus Element Out6/1

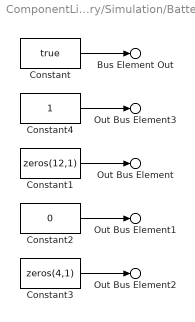
== system ComponentLibrary/Simulation/Battery ==
  Constant : Constant  Value=true  OutDataTypeStr=boolean
  Constant1 : Constant  Value=zeros(12,1)
  Constant2 : Constant  Value=0
  Constant3 : Constant  Value=zeros(4,1)
  Constant4 : Constant
  Bus Element Out : Outport  PortName=OutBus  Element=dataGood
  Out Bus Element3 : Outport  PortName=OutBus  Element=stateOfCharge
  Out Bus Element : Outport  PortName=OutBus  Element=voltage
  Out Bus Element1 : Outport  PortName=OutBus  Element=current
  Out Bus Element2 : Outport  PortName=OutBus  Element=temperature
  wires:
  Constant/1 -> Bus Element Out/1
  Constant3/1 -> Out Bus Element2/1
  Constant2/1 -> Out Bus Element1/1
  Constant1/1 -> Out Bus Element/1
  Constant4/1 -> Out Bus Element3/1

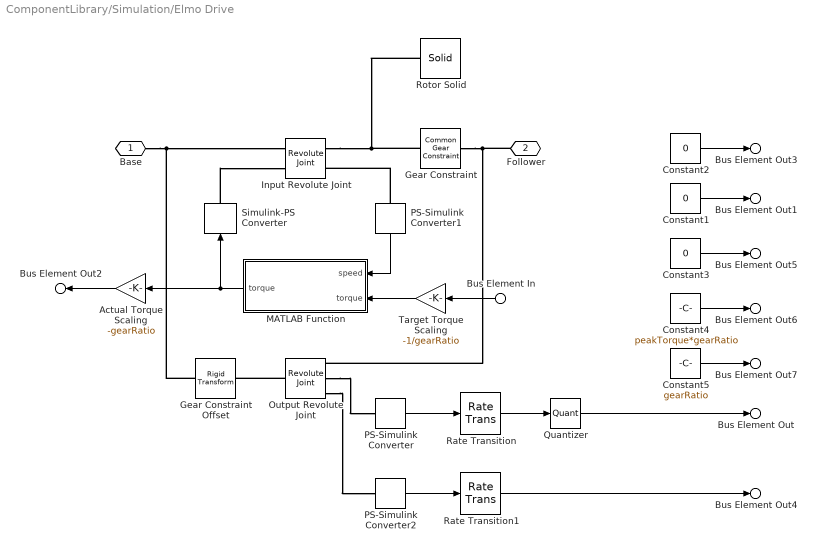
== system ComponentLibrary/Simulation/Elmo Drive ==
  Bus Element In : Inport  PortName=InBus  Element=torque
  Actual Torque Scaling : Gain  Gain=-gearRatio
  Constant1 : Constant  Value=0
  Constant2 : Constant  Value=0  OutDataTypeStr=uint16
  Constant3 : Constant  Value=0
  Constant4 : Constant  Value=peakTorque*gearRatio
  Constant5 : Constant  Value=gearRatio
  Gear Constraint : sm_lib/Gears and Couplings/Gears/Common Gear Constraint  GearType=External  SpecificationType=CenterDistanceRatio  CenterDistance=1e-6  CenterDistanceUnits=m  GearRatio=gearRatio  BaseGearRadius=10.0  BaseGearRadiusUnits=cm  FollGearRadius=10.0  FollGearRadiusUnits=cm  AssemblyGearRotation=Free
      settings: SourceProductName=Simscape Multibody  SourceProductBaseCode=MS
  Gear Constraint Offset : sm_lib/Frames and Transforms/Rigid Transform  TranslationMethod=StandardAxis  TranslationStandardOffset=1e-6  TranslationLengthUnit=m  TranslationStandardAxis=+Y  TranslationCartesianOffset=[0 0 0]  TranslationROffset=0  TranslationROffsetUnits=m  TranslationZOffset=0  TranslationZOffsetUnits=m  TranslationThetaOffset=0  TranslationThetaOffsetUnits=deg  RotationMethod=None  RotationAngleUnits=deg  RotationStandardAxis=+Z  RotationAngle=0.0  RotationArbitraryAxis=[0 0 1]  FollAlignAxisA=+X  BaseAlignAxisA=+Y  FollAlignAxisB=+Y  BaseAlignAxisB=+Z  RotationSequenceAxes=FollowerAxes  RotationSequence=XYX  RotationSequenceAngles=[0 0 0]  RotationSequenceAnglesUnits=deg  RotationMatrix=[1 0 0; 0 1 0; 0 0 1]
  Input Revolute Joint : sm_lib/Joints/Revolute Joint  SenseConstraintForce=off  SenseConstraintForceX=off  SenseConstraintForceY=off  SenseConstraintForceZ=off  SenseConstraintTorque=off  SenseConstraintTorqueX=off  SenseConstraintTorqueY=off  SenseConstraintTorqueZ=off  SenseTotalForce=off  SenseTotalForceX=off  SenseTotalForceY=off  SenseTotalForceZ=off  SenseTotalTorque=off  SenseTotalTorqueX=off  SenseTotalTorqueY=off  SenseTotalTorqueZ=off  CompositeWrenchDir=FollowerOnBase  CompositeWrenchFrame=BaseFrame  EquilibriumPosition=0  EquilibriumPositionUnits=rad  SpringStiffness=0  SpringStiffnessUnits=N*m/rad  DampingCoefficient=0  DampingCoefficientUnits=N*m/(rad/s)  TorqueActuationMode=InputTorque  MotionActuationMode=ComputedMotion  SensePosition=off  SenseVelocity=on  SenseAcceleration=off  SenseTorqueForce=off  PositionTargetSpecify=off  PositionTargetPriority=High  PositionTargetValue=0  PositionTargetValueUnits=deg  VelocityTargetSpecify=off  VelocityTargetPriority=High  VelocityTargetValue=0  VelocityTargetValueUnits=rad/s
  MATLAB Function : MATLAB Function  TreatAsAtomicUnit=on
  Output Revolute Joint : sm_lib/Joints/Revolute Joint  SenseConstraintForce=off  SenseConstraintForceX=off  SenseConstraintForceY=off  SenseConstraintForceZ=off  SenseConstraintTorque=off  SenseConstraintTorqueX=off  SenseConstraintTorqueY=off  SenseConstraintTorqueZ=off  SenseTotalForce=off  SenseTotalForceX=off  SenseTotalForceY=off  SenseTotalForceZ=off  SenseTotalTorque=off  SenseTotalTorqueX=off  SenseTotalTorqueY=off  SenseTotalTorqueZ=off  CompositeWrenchDir=FollowerOnBase  CompositeWrenchFrame=BaseFrame  EquilibriumPosition=0  EquilibriumPositionUnits=rad  SpringStiffness=0  SpringStiffnessUnits=N*m/rad  DampingCoefficient=1  DampingCoefficientUnits=N*m/(rad/s)  TorqueActuationMode=NoTorque  MotionActuationMode=ComputedMotion  SensePosition=on  SenseVelocity=on  SenseAcceleration=off  SenseTorqueForce=off  PositionTargetSpecify=on  PositionTargetPriority=High  PositionTargetValue=initialPosition  PositionTargetValueUnits=rad  VelocityTargetSpecify=on  VelocityTargetPriority=High  VelocityTargetValue=initialVelocity  VelocityTargetValueUnits=rad/s
  PS-Simulink Converter : nesl_utility/PS-Simulink Converter  PhysicalDomain=network_engine_domain  SubClassName=ps_output  LeftPortType=input  RightPortType=output  PseudoPeriodic=off  Frequencies=[]  Unit=rad  AffineConversion=off
  PS-Simulink Converter1 : nesl_utility/PS-Simulink Converter  PhysicalDomain=network_engine_domain  SubClassName=ps_output  LeftPortType=input  RightPortType=output  PseudoPeriodic=off  Frequencies=[]  Unit=rad/s  AffineConversion=off
  PS-Simulink Converter2 : nesl_utility/PS-Simulink Converter  PhysicalDomain=network_engine_domain  SubClassName=ps_output  LeftPortType=input  RightPortType=output  PseudoPeriodic=off  Frequencies=[]  Unit=rad/s  AffineConversion=off
  Quantizer : Quantizer  QuantizationInterval=(2*pi)/(encoderResolution*gearRatio)
  Rate Transition : RateTransition  Deterministic=off  InitialCondition=initialPosition  OutPortSampleTimeOpt=Inherit
  Rate Transition1 : RateTransition  Deterministic=off  InitialCondition=initialPosition  OutPortSampleTimeOpt=Inherit
  Rotor Solid : sm_lib/Body Elements/Solid  InertiaType=Custom  Mass=0  MassUnits=kg  CenterOfMass=[0; 0; 0]  CenterOfMassUnits=m  MomentsOfInertia=[0; 0; rotorInertia]  MomentsOfInertiaUnits=kg*m^2  ProductsOfInertia=[0; 0; 0]  ProductsOfInertiaUnits=kg*m^2  DensityBased=on  Density=1000  DensityUnits=kg/m^3  DoExposeReferenceFrame=on  SerializedFrames=<Frames/>  GraphicType=None  MarkerShape=Sphere  MarkerSize=10  GraphicVisPropType=SimpleVisualProperties  GraphicDiffuseColor=[0.5 0.5 0.5]  GraphicSpecularColor=[0.5 0.5 0.5 1.0]  GraphicAmbientColor=[0.15 0.15 0.15 1.0]  GraphicEmissiveColor=[0.0 0.0 0.0 1.0]  GraphicShininess=75  GraphicOpacity=1.0  GeometryShape=Cylinder  RectangleSize=[1 1]  RectangleSizeUnits=m  BrickDimensions=[1 1 1]  BrickDimensionUnits=m  CylinderRadius=1  CylinderRadiusUnits=m  CylinderLength=1  CylinderLengthUnits=m  SphereRadius=1  SphereRadiusUnits=m  EllipsoidRadii=[1 1 1]  EllipsoidRadiiUnits=m  ExtrusionCrossSection=[1 1; -1 1; -1 -1; 1 -1]  ExtrusionCrossSectionUnits=m  ExtrusionLength=1  ExtrusionLengthUnits=m  PolygonNumSides=3  PolygonOuterRadius=1  PolygonOuterRadiusUnits=m  ExtGeomFileType=STEP  ExtGeomFileUnits=m  RevolutionCrossSection=[1 1; 1 -1; 2 -1; 2 1]  RevolutionCrossSectionUnits=m  RevolutionExtent=Full  RevolutionAngle=180  RevolutionAngleUnits=deg
  Simulink-PS Converter : nesl_utility/Simulink-PS Converter  PhysicalDomain=network_engine_domain  SubClassName=ps_input  LeftPortType=input  RightPortType=output  PseudoPeriodic=off  Frequencies=[]  NoiseDistribution=none  NoiseParameters=[]  Unit=N*m  AffineConversion=off  FilteringAndDerivatives=zero  SimscapeFilterOrder=1  InputFilterTimeConstant=0.001  UdotUserProvided=1
  Target Torque Scaling : Gain  Gain=-1/gearRatio
  Base : PMIOPort  Port=1  Side=Left
  Follower : PMIOPort  Port=2  Side=Right
  Bus Element Out3 : Outport  PortName=OutBus  Element=statusWord
  Bus Element Out : Outport  PortName=OutBus  Element=position
  Bus Element Out4 : Outport  PortName=OutBus  Element=velocity
  Bus Element Out2 : Outport  PortName=OutBus  Element=torque
  Bus Element Out1 : Outport  PortName=OutBus  Element=driveTemperature
  Bus Element Out5 : Outport  PortName=OutBus  Element=dcLinkVoltage
  Bus Element Out6 : Outport  PortName=OutBus  Element=torqueLimit
  Bus Element Out7 : Outport  PortName=OutBus  Element=gearRatio
  wires:
  Rate Transition/1 -> Quantizer/1
  PS-Simulink Converter/1 -> Rate Transition/1
  Quantizer/1 -> Bus Element Out/1
  Bus Element In/1 -> Target Torque Scaling/1
  MATLAB Function/1(torque) -> Actual Torque Scaling/1, Simulink-PS Converter/1
  PS-Simulink Converter1/1 -> MATLAB Function/1(speed)
  Target Torque Scaling/1 -> MATLAB Function/2("torque ")
  Constant2/1 -> Bus Element Out3/1
  Constant1/1 -> Bus Element Out1/1
  Constant3/1 -> Bus Element Out5/1
  Constant4/1 -> Bus Element Out6/1
  Actual Torque Scaling/1 -> Bus Element Out2/1
  Constant5/1 -> Bus Element Out7/1
  Rate Transition1/1 -> Bus Element Out4/1
  PS-Simulink Converter2/1 -> Rate Transition1/1
  connections:
  Output Revolute Joint/RConn2 -- PS-Simulink Converter/LConn1
  Output Revolute Joint/LConn1 -- Gear Constraint Offset/RConn1
  Gear Constraint/RConn1 -- Follower/RConn1 -- Output Revolute Joint/RConn1
  Input Revolute Joint/RConn1 -- Gear Constraint/LConn1 -- Rotor Solid/RConn1
  PS-Simulink Converter1/LConn1 -- Input Revolute Joint/RConn2
  Simulink-PS Converter/RConn1 -- Input Revolute Joint/LConn2
  Gear Constraint Offset/LConn1 -- Base/RConn1 -- Input Revolute Joint/LConn1
  Output Revolute Joint/RConn3 -- PS-Simulink Converter2/LConn1
